simulink model "jacobitest"  (R2023b)
settings: Solver=VariableStepAuto  StartTime=0.0  StopTime=10.0  RelTol=1e-3
libraries: robotmaniplib x9
settings Model: Creator=shobhit  LastModifiedBy=shobhit

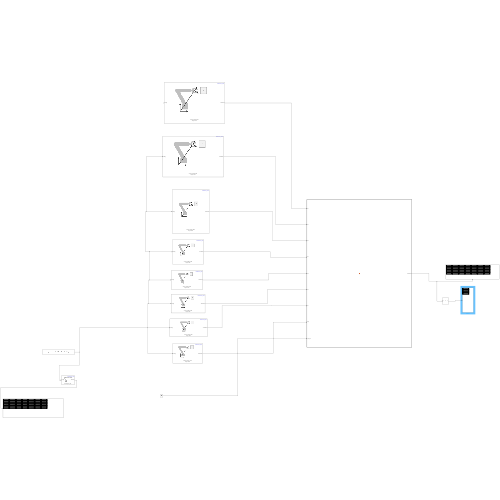
[thumbnail: Simulink's stored preview of the top-level diagram]
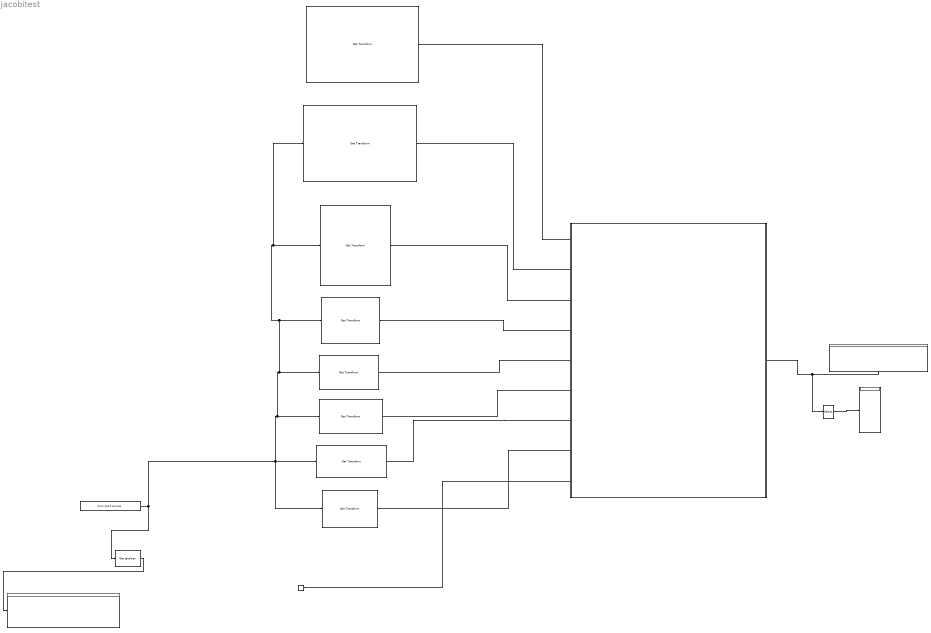
== system jacobitest ==
  Constant : Constant  Value=[0 0 0 -pi/2 0 pi/2 pi/4]
  Constant1 : Constant  Value=8
  Display : Display
  Display1 : Display
  Display2 : Display
  Get Jacobian : robotmaniplib/Get Jacobian  RigidBodyTree=frankarobot_mdh  EndEffector=Gripper_TCP  SimulateUsing=Interpreted execution
  Get Transform : robotmaniplib/Get Transform  RigidBodyTree=frankarobot_mdh  SourceBody=Franka_link7  TargetBody=base  SimulateUsing=Interpreted execution
  Get Transform1 : robotmaniplib/Get Transform  RigidBodyTree=frankarobot_mdh  SourceBody=Franka_link6  TargetBody=base  SimulateUsing=Interpreted execution
  Get Transform2 : robotmaniplib/Get Transform  RigidBodyTree=frankarobot_mdh  SourceBody=Franka_link5  TargetBody=base  SimulateUsing=Interpreted execution
  Get Transform3 : robotmaniplib/Get Transform  RigidBodyTree=frankarobot_mdh  SourceBody=Franka_link4  TargetBody=base  SimulateUsing=Interpreted execution
  Get Transform4 : robotmaniplib/Get Transform  RigidBodyTree=frankarobot_mdh  SourceBody=Franka_link3  TargetBody=base  SimulateUsing=Interpreted execution
  Get Transform5 : robotmaniplib/Get Transform  RigidBodyTree=frankarobot_mdh  SourceBody=Franka_link2  TargetBody=base  SimulateUsing=Interpreted execution
  Get Transform6 : robotmaniplib/Get Transform  RigidBodyTree=frankarobot_mdh  SourceBody=Franka_link1  TargetBody=base  SimulateUsing=Interpreted execution
  Get Transform7 : robotmaniplib/Get Transform  RigidBodyTree=frankarobot_mdh  SourceBody=Gripper_TCP  TargetBody=base  SimulateUsing=Interpreted execution
  MATLAB Function : MATLAB Function  TreatAsAtomicUnit=on
  Selector : Selector  NumberOfDimensions=2  InputPortWidth=3  IndexOptions=Index vector (dialog),Index vector (dialog)  Indices=[1 2 3 4],7  OutputSizes=5,1
  wires:
  Constant/1 -> Get Jacobian/1, Get Transform3/1, Get Transform5/1, Get Transform4/1, Get Transform2/1, Get Transform1/1, Get Transform7/1, Get Transform/1
  Get Jacobian/1 -> Display/1
  Get Transform7/1 -> MATLAB Function/8(T0tcp)
  Get Transform/1 -> MATLAB Function/7(T07)
  Get Transform1/1 -> MATLAB Function/6(T06)
  Get Transform2/1 -> MATLAB Function/5(T05)
  Get Transform3/1 -> MATLAB Function/4(T04)
  Get Transform4/1 -> MATLAB Function/3(T03)
  Get Transform5/1 -> MATLAB Function/2(T02)
  Get Transform6/1 -> MATLAB Function/1(T01)
  Constant1/1 -> MATLAB Function/9(to_ith_link)
  MATLAB Function/1(Jacobimatrix) -> Selector/1, Display1/1
  Selector/1 -> Display2/1

== matlab function jacobitest/MATLAB Function ==
  data: T01 input; Jacobimatrix output; T02 input; T03 input; T04 input; T05 input; T06 input; T07 input; T0tcp input; to_ith_link input
function Jacobimatrix = fcn(T01,T02,T03,T04,T05,T06,T07,T0tcp,to_ith_link)

%Array of transformation matrices 
T = {T01,T02,T03,T04,T05,T06,T07,T0tcp};

numJoints = 7; % Number of joints
J = zeros(6, numJoints); % Initialize Jacobian matrix with zeros
    if to_ith_link == 8 
        T_end_effector = T0tcp;
    else
    % Compute the transformation to the end-effector or to_ith_link
    T_end_effector = T07;
    end
    
    end_effector_position = T_end_effector(1:3, 4);

    for i = 1:to_ith_link-1
        % Get the transformation matrix from the base frame to the ith joint
        T_i = T{i};

        % Extract the z-axis of the ith joint in base frame coordinates
        z_i = T_i(1:3, 1:3) * [0; 0; 1];

        % Position of the ith joint in base frame coordinates
        d_i = T_i(1:3, 4);

        % Linear velocity contribution: cross product of z-axis with the vector from joint i to the end-effector
        Jv_i = cross(z_i, (end_effector_position - d_i));

        % Angular velocity contribution: simply the z-axis for revolute joints
        Jw_i = z_i;

        % Fill in the ith column of the Jacobian matrix for joint i
        J(1:3, i) = Jv_i; % Upper part for linear velocity
        J(4:6, i) = Jw_i; % Lower part for angular velocity
    end

    % Columns of Jacobian corresponding to joints beyond to_ith_link are already initialized to zero
    Jacobimatrix = J;
end
